simulink model "Cable_Angle_verification"  (R2019b)
settings: Solver=VariableStepAuto  StartTime=0.0  StopTime=10.0  RelTol=1e-3
undefined symbols (not defined in the file): d, r
settings Model: Creator=zceeash  LastModifiedBy=arund

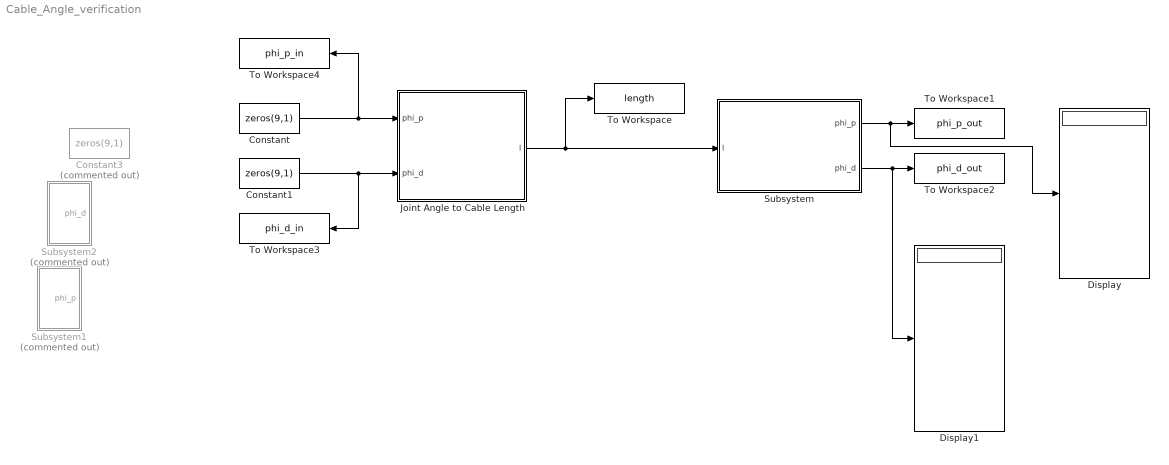
== system Cable_Angle_verification ==
  Constant : Constant  Value=zeros(9,1)
  Constant1 : Constant  Value=zeros(9,1)
  Constant3 : Constant  Commented=on  Value=zeros(9,1)
  Display : Display
  Display1 : Display
  Joint Angle to Cable Length : MATLAB Function  TreatAsAtomicUnit=on
  Subsystem : Subsystem
  Subsystem1 : Subsystem  Commented=on
  Subsystem2 : Subsystem  Commented=on
  To Workspace : ToWorkspace  VariableName=length  SampleTime=-1
  To Workspace1 : ToWorkspace  VariableName=phi_p_out  SampleTime=-1
  To Workspace2 : ToWorkspace  VariableName=phi_d_out  SampleTime=-1
  To Workspace3 : ToWorkspace  VariableName=phi_d_in  SampleTime=-1
  To Workspace4 : ToWorkspace  VariableName=phi_p_in  SampleTime=-1
  wires:
  Joint Angle to Cable Length/1(l) -> Subsystem/1(l), To Workspace/1
  Constant1/1 -> To Workspace3/1, Joint Angle to Cable Length/2(phi_d)
  Subsystem/1(phi_p) -> Display/1, To Workspace1/1
  Subsystem/2(phi_d) -> Display1/1, To Workspace2/1
  Constant/1 -> To Workspace4/1, Joint Angle to Cable Length/1(phi_p)

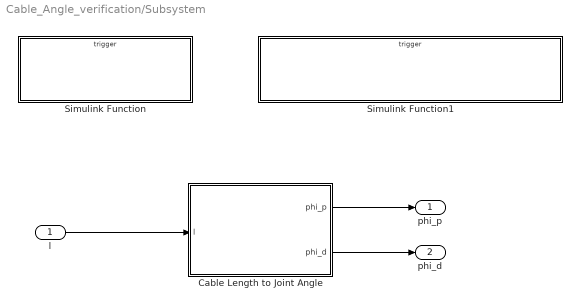
== system Cable_Angle_verification/Subsystem ==
  l : Inport
  " Cable Length to Joint Angle" : MATLAB Function  TreatAsAtomicUnit=on
  Simulink Function : Subsystem  TreatAsAtomicUnit=on
  Simulink Function1 : Subsystem  TreatAsAtomicUnit=on
  phi_p : Outport
  phi_d : Outport  Port=2
  wires:
  l/1 -> " Cable Length to Joint Angle"/1(l)
  " Cable Length to Joint Angle"/1(phi_p) -> phi_p/1
  " Cable Length to Joint Angle"/2(phi_d) -> phi_d/1

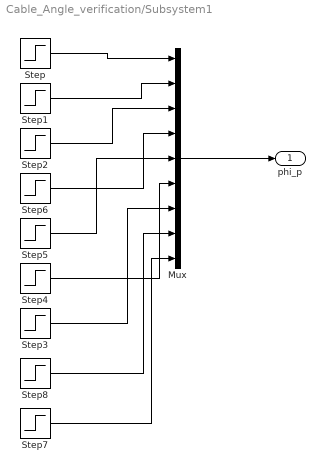
== system Cable_Angle_verification/Subsystem1 ==
  Mux : Mux  Inputs=9
  Step : Step  After=0.1  SampleTime=0
  Step{1..8} (8 alike) : Step  After=0  SampleTime=0
  phi_p : Outport
  wires:
  Mux/1 -> phi_p/1
  Step/1 -> Mux/1
  Step1/1 -> Mux/2
  Step2/1 -> Mux/3
  Step6/1 -> Mux/4
  Step5/1 -> Mux/5
  Step4/1 -> Mux/6
  Step3/1 -> Mux/7
  Step8/1 -> Mux/8
  Step7/1 -> Mux/9

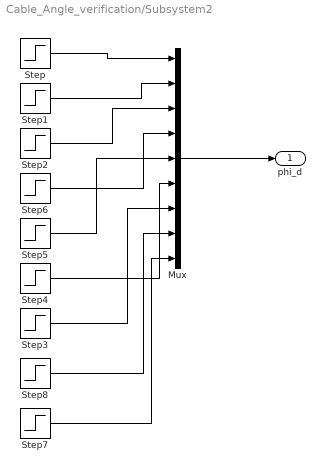
== system Cable_Angle_verification/Subsystem2 ==
  Mux : Mux  Inputs=9
  Step{,1..8} (9 alike) : Step  After=0  SampleTime=0
  phi_d : Outport
  wires:
  Mux/1 -> phi_d/1
  Step/1 -> Mux/1
  Step1/1 -> Mux/2
  Step2/1 -> Mux/3
  Step6/1 -> Mux/4
  Step5/1 -> Mux/5
  Step4/1 -> Mux/6
  Step3/1 -> Mux/7
  Step8/1 -> Mux/8
  Step7/1 -> Mux/9

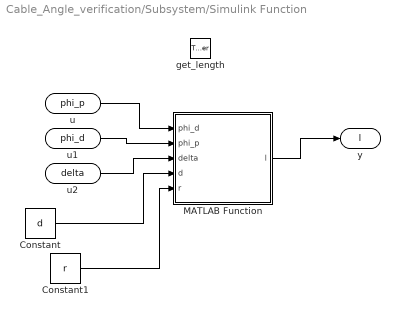
== system Cable_Angle_verification/Subsystem/Simulink Function ==
  get_length : TriggerPort  TriggerType=function-call  IsSimulinkFunction=on  FunctionName=get_length  FunctionVisibility=scoped  VariantControl=(inherit)
  Constant : Constant  Value=d
  Constant1 : Constant  Value=r
  MATLAB Function : MATLAB Function  TreatAsAtomicUnit=on
  u : ArgIn  DisableCoverage=on  ArgumentName=phi_p
  u1 : ArgIn  DisableCoverage=on  Port=2  ArgumentName=phi_d
  u2 : ArgIn  DisableCoverage=on  Port=3  ArgumentName=delta
  y : ArgOut  DisableCoverage=on  ArgumentName=l
  wires:
  MATLAB Function/1(l) -> y/1
  u/1 -> MATLAB Function/1(phi_d)
  u1/1 -> MATLAB Function/2(phi_p)
  u2/1 -> MATLAB Function/3(delta)
  Constant/1 -> MATLAB Function/4(d)
  Constant1/1 -> MATLAB Function/5(r)

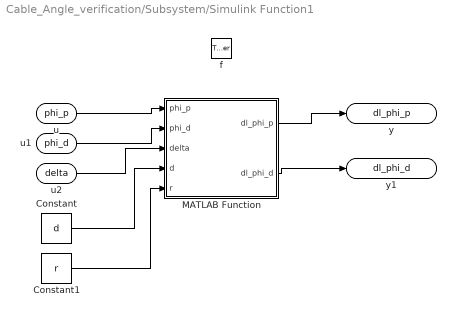
== system Cable_Angle_verification/Subsystem/Simulink Function1 ==
  f : TriggerPort  TriggerType=function-call  IsSimulinkFunction=on  FunctionName=get_partial_diff  FunctionVisibility=scoped  VariantControl=(inherit)
  Constant : Constant  Value=d
  Constant1 : Constant  Value=r
  MATLAB Function : MATLAB Function  TreatAsAtomicUnit=on
  u : ArgIn  DisableCoverage=on  ArgumentName=phi_p
  u1 : ArgIn  DisableCoverage=on  Port=2  ArgumentName=phi_d
  u2 : ArgIn  DisableCoverage=on  Port=3  ArgumentName=delta
  y : ArgOut  DisableCoverage=on  ArgumentName=dl_phi_p
  y1 : ArgOut  DisableCoverage=on  Port=2  ArgumentName=dl_phi_d
  wires:
  MATLAB Function/1(dl_phi_p) -> y/1
  u/1 -> MATLAB Function/1(phi_p)
  u1/1 -> MATLAB Function/2(phi_d)
  u2/1 -> MATLAB Function/3(delta)
  MATLAB Function/2(dl_phi_d) -> y1/1
  Constant/1 -> MATLAB Function/4(d)
  Constant1/1 -> MATLAB Function/5(r)

== matlab function Cable_Angle_verification/Joint Angle to Cable Length ==
  data: l output; phi_p input; phi_d input
function l = fcn(phi_p,phi_d)
N=9;
d=23/2/1000;
r=20.5/1000;
l=zeros(3*N,1);
% Calculate transformation matrices
A=cell(N,1);
for n=1:N
    s_p=sin(phi_p(n));
    s_d=sin(phi_d(n));
    c_p=cos(phi_p(n));
    c_d=cos(phi_d(n));
    A{n}=[ c_p        0     s_p        s_p*d;...
           s_d*s_p   c_d   -s_d*c_p   -d*s_d*c_p ;...
           -c_d*s_p   s_d    c_p*c_d    d*(c_p*c_d+1);...
             0         0      0          1];
end
% Calculate the length of cable between joints
for k=1:3*N
    l_k = 0;
    % The link at which cable k terminates
    M = floor((k-1)/3)+1;
    for n=1:M
        % Calculate the angular position of the hole on distal and proximal
        % discs
        if rem(n,2)==0
            delta_p=((120/(N+1))*(M)+120*(k-1)+87);
            delta_d=((120/(N+1))*(M)+120*(k-1)-3);
        else
            delta_p=((120/(N+1))*(M)+120*(k-1)-3);
            delta_d=((120/(N+1))*(M)+120*(k-1)+87);
        end
        % Calculate hole position vector on distal and proximal discs
        c_delta_p=cosd(delta_p);
        s_delta_p=sind(delta_p);
        c_delta_d=cosd(delta_d);
        s_delta_d=sind(delta_d);
        H_p=[r*c_delta_p;r*s_delta_p;0;1];
        H_d=[r*c_delta_d;r*s_delta_d;0;1];
        % Get the length of cable between the proximal and distal disc at
        % joint n
        trans_H_p=A{n}*H_p;
        l_k_n=trans_H_p(1:3)-H_d(1:3);
        l_k = l_k + norm(l_k_n);
    end
    l(k)=l_k;
end

== matlab function Cable_Angle_verification/Subsystem/ Cable Length to Joint Angle ==
  data: phi_p output; l input; phi_d output
function [phi_p,phi_d] = fcn(l)
N=9;
d=23/2/1000;
r=20.5/1000;
error_tol=1/1000;
phi_d=zeros(N,1);
phi_p=zeros(N,1);
% Numerical iteration to find solution
for n=1:N
    % Get delta
    if rem(n,2)==0
        delta=[(12*(round(((3*n)-1)/3)+1)+120*((3*n)-1)+90)*pi/180;...
               (12*(round(((3*n-1)-1)/3)+1)+120*((3*n-1)-1)+90)*pi/180;...
               (12*(round(((3*n-2)-1)/3)+1)+120*((3*n-2)-1)+90)*pi/180];
    else
        delta = [(12*(round(((3*n)-1)/3)+1)+120*((3*n)-1))*pi/180; ...
                (12*(round(((3*n-1)-1)/3)+1)+120*((3*n-1)-1))*pi/180; ...
                (12*(round(((3*n-2)-1)/3)+1)+120*((3*n-2)-1))*pi/180];
    end

   l_d=l(3*n-2:3*n);
   l_d=l_d/N;
   
   phi_j=[0;0];
   
   for j=0:500
       % Calculate l_j
       l_3n_0=get_length(phi_j(1),phi_j(2),delta(1));
       l_3n_1=get_length(phi_j(1),phi_j(2),delta(2));
       l_3n_2=get_length(phi_j(1),phi_j(2),delta(3));
       l_j=[l_3n_0;...
            l_3n_1;...
            l_3n_2];
       % Calculate error
       delta_l=l_d-l_j;
       % Check if the error is within tolerance
       if (delta_l(1)<=error_tol) && (delta_l(2)<=error_tol) && (delta_l(3)<=error_tol)
           phi_d(n)=phi_j(1);
           phi_p(n)=phi_j(2);
           break;
       end
       % Calculate the Jacobian         
       [J_1_1 J_1_2] = get_partial_diff(phi_j(1),phi_j(2),delta(1));
       [J_2_1 J_2_2] = get_partial_diff(phi_j(1),phi_j(2),delta(2));
       [J_3_1 J_3_2] = get_partial_diff(phi_j(1),phi_j(2),delta(3));
       J=[[J_1_1 J_1_2];...
          [J_2_1 J_2_2];...
          [J_3_1 J_3_2]];
       J_inv=pinv(J);
       %Calculate error
       delta_phi= J_inv*delta_l;
       % Use error to estimate delta_theta
       phi_j=phi_j+delta_phi;
       
       if j==10000
           phi_d(n)=NaN;
           phi_p(n)=NaN;
       end
   end
end

== matlab function Cable_Angle_verification/Subsystem/Simulink Function/MATLAB Function ==
  data: phi_d input; l output; phi_p input; delta input; d input; r input
function l = fcn(phi_d,phi_p,delta,d,r)
l = sqrt((d*sin(phi_d)+r*cos(phi_d)*cos(delta)-r*cos(delta))^2 + ...
         (r*cos(delta)*sin(phi_p)*sin(phi_d)+r*cos(phi_p)*sin(delta)-d*sin(phi_p)*cos(phi_d)-r*sin(delta))^2 + ...
         (r*sin(phi_p)*sin(delta)-r*cos(delta)*cos(phi_p)*sin(phi_d)+d*cos(phi_p)*cos(phi_d)+d)^2);

== matlab function Cable_Angle_verification/Subsystem/Simulink Function1/MATLAB Function ==
  data: phi_p input; dl_phi_p output; phi_d input; delta input; dl_phi_d output; d input; r input
function [dl_phi_p,dl_phi_d] = fcn(phi_p,phi_d,delta,d,r)
dl_phi_p =(2*(r*cos(phi_p)*sin(delta) - d*cos(phi_d)*sin(phi_p) + ... 
           r*cos(delta)*sin(phi_d)*sin(phi_p))*(d + ... 
           d*cos(phi_d)*cos(phi_p) + r*sin(delta)*sin(phi_p) - ...
           r*cos(delta)*cos(phi_p)*sin(phi_d)) + ... 
           2*(d*cos(phi_d)*cos(phi_p) + r*sin(delta)*sin(phi_p) - ...
           r*cos(delta)*cos(phi_p)*sin(phi_d))*(r*sin(delta) + ...
           d*cos(phi_d)*sin(phi_p) - r*cos(phi_p)*sin(delta) - ... 
           r*cos(delta)*sin(phi_d)*sin(phi_p)))/(2*((d + ...
           d*cos(phi_d)*cos(phi_p) + r*sin(delta)*sin(phi_p) - ... 
           r*cos(delta)*cos(phi_p)*sin(phi_d))^2 + (d*sin(phi_d) - ... 
           r*cos(delta) + r*cos(delta)*cos(phi_d))^2 + (r*sin(delta) + ... 
           d*cos(phi_d)*sin(phi_p) - r*cos(phi_p)*sin(delta) - ... 
           r*cos(delta)*sin(phi_d)*sin(phi_p))^2)^(1/2));
       
dl_phi_d = -(2*(d*cos(phi_p)*sin(phi_d) + ...
             r*cos(delta)*cos(phi_d)*cos(phi_p))*...
             (d + d*cos(phi_d)*cos(phi_p) + ... 
             r*sin(delta)*sin(phi_p) - ...
             r*cos(delta)*cos(phi_p)*sin(phi_d)) - 2*(d*cos(phi_d) - ...
             r*cos(delta)*sin(phi_d))*(d*sin(phi_d) - r*cos(delta) + ...
             r*cos(delta)*cos(phi_d)) + 2*(d*sin(phi_d)*sin(phi_p) + ...
             r*cos(delta)*cos(phi_d)*sin(phi_p))*(r*sin(delta) + ...
             d*cos(phi_d)*sin(phi_p) - r*cos(phi_p)*sin(delta) - ...
             r*cos(delta)*sin(phi_d)*sin(phi_p)))/(2*((d + d*cos(phi_d)*cos(phi_p) + ... 
             r*sin(delta)*sin(phi_p) - ...
             r*cos(delta)*cos(phi_p)*sin(phi_d))^2 + (d*sin(phi_d) - ...
             r*cos(delta) + r*cos(delta)*cos(phi_d))^2 + (r*sin(delta) + ...
             d*cos(phi_d)*sin(phi_p) - r*cos(phi_p)*sin(delta) - ...
             r*cos(delta)*sin(phi_d)*sin(phi_p))^2)^(1/2));
